simulink model "Innerloop_joystick_PIL_block"  (R2015a)
settings: Solver=ode45  StartTime=0.0  StopTime=100  FixedStep=0.01  RelTol=1e-3
undefined symbols (not defined in the file or in its folder): kdp, kdps, kdt, kdz, kpp, kpps, kpt, kpz
libraries: vrlib x1
settings Model: Creator=abdelrazzak.merheb  LastModifiedBy=flying
settings DataIOCC: SignalLoggingSaveFormat=ModelDataLogs
settings OptimizationCC: ExpressionDepthLimit=2147483647
settings DebuggingCC: UnderspecifiedInitializationDetection=Classic  MergeDetectMultiDrivingBlocksExec=none  SolverPrmCheckMsg=warning  FcnCallInpInsideContextMsg=UseLocalSettings  StateNameClashWarn=warning
settings GRTTargetCC: CombineOutputUpdateFcns=off  GRTInterface=on

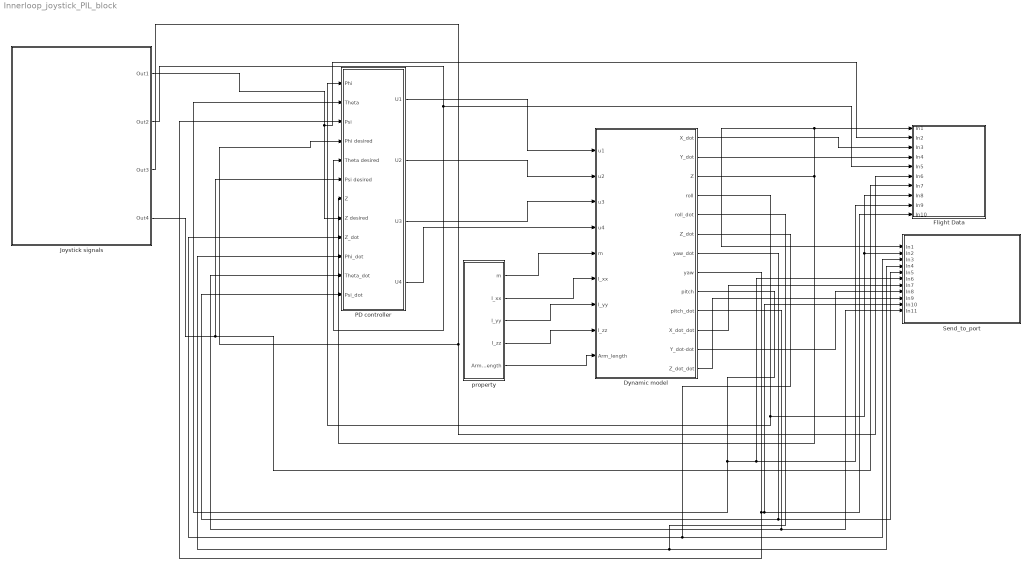
== system Innerloop_joystick_PIL_block ==
  Dynamic model : Subsystem
  Flight Data : Subsystem
  Joystick signals : Subsystem
  PD controller : Subsystem
  Send_to_port : Subsystem
  "property " : Subsystem
  wires:
  Dynamic model/9(pitch) -> PD controller/2(Theta), Flight Data/9(In9), Send_to_port/6(In6)
  Dynamic model/3(Z) -> PD controller/7(Z), Send_to_port/1(In1), Flight Data/1(In1)
  Dynamic model/4(roll) -> PD controller/1(Phi), Flight Data/8(In8), Send_to_port/2(In2)
  Dynamic model/6(Z_dot) -> Send_to_port/3(In3), PD controller/9(Z_dot)
  Dynamic model/5(roll_dot) -> Send_to_port/4(In4), PD controller/10(Phi_dot)
  Dynamic model/10(pitch_dot) -> PD controller/11(Theta_dot), Send_to_port/11(In11)
  Dynamic model/7(yaw_dot) -> PD controller/12("Psi_dot "), Send_to_port/5(In5)
  Dynamic model/8(yaw) -> PD controller/3(Psi), Flight Data/10(In10), Send_to_port/10(In10)
  Dynamic model/11(X_dot_dot) -> Send_to_port/7(In7)
  Dynamic model/12(Y_dot-dot) -> Send_to_port/8(In8)
  Dynamic model/13(Z_dot_dot) -> Send_to_port/9(In9)
  Joystick signals/4(Out4) -> Flight Data/7(In7), PD controller/6(Psi desired)
  Joystick signals/3(Out3) -> Flight Data/6(In6), PD controller/4(Phi desired)
  Joystick signals/2(Out2) -> PD controller/5(Theta desired), Flight Data/5(In5)
  Joystick signals/1(Out1) -> Flight Data/2(In2), PD controller/8(Z desired)
  Dynamic model/1("X_dot ") -> Flight Data/3(In3)
  Dynamic model/2(Y_dot) -> Flight Data/4(In4)
  "property "/5("Arm_length ") -> Dynamic model/9(Arm_length)
  "property "/4(I_zz) -> Dynamic model/8(I_zz)
  "property "/3(I_yy) -> Dynamic model/7(I_yy)
  "property "/2(I_xx) -> Dynamic model/6(I_xx)
  "property "/1(m) -> Dynamic model/5(m)
  PD controller/2(U2) -> Dynamic model/2(u2)
  PD controller/3(U3) -> Dynamic model/3(u3)
  PD controller/1(U1) -> Dynamic model/1(u1)
  PD controller/4(U4) -> Dynamic model/4(u4)

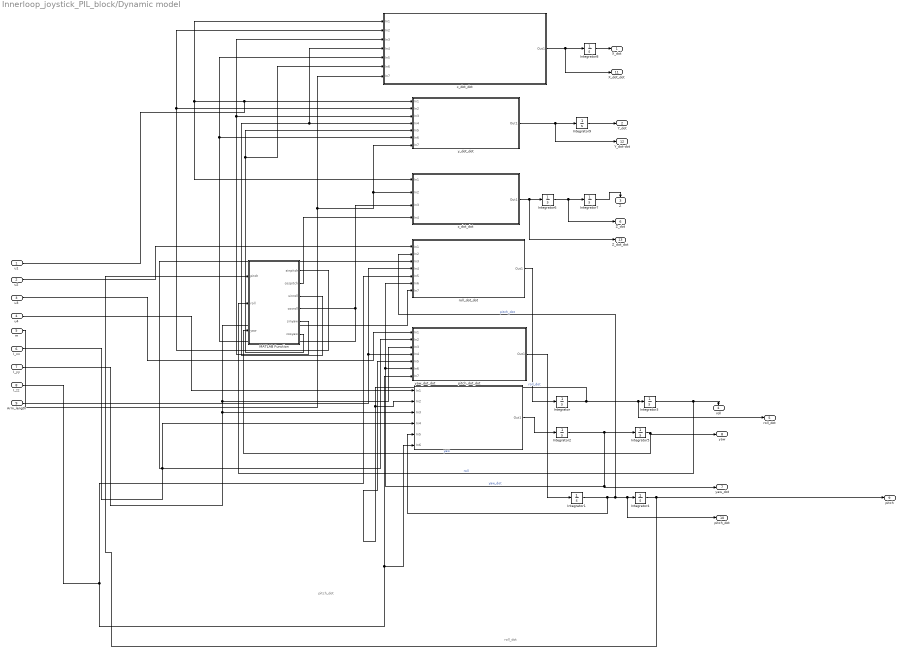
== system Innerloop_joystick_PIL_block/Dynamic model ==
  note: pitch_dot
  note: roll_dot
  u1 : Inport
  u2 : Inport  Port=2
  u3 : Inport  Port=3
  u4 : Inport  Port=4
  m : Inport  Port=5
  I_xx : Inport  Port=6
  I_yy : Inport  Port=7
  I_zz : Inport  Port=8
  Arm_length : Inport  Port=9
  Integrator{,1..9} (10 alike) : Integrator
  MATLAB Function : MATLAB Function  TreatAsAtomicUnit=on
  pitch_dot_dot : Subsystem
  roll_dot_dot : Subsystem
  x_dot_dot : Subsystem
  y_dot_dot : Subsystem
  yaw_dot_dot : Subsystem
  z_dot_dot : Subsystem
  "X_dot " : Outport
  Y_dot : Outport  Port=2
  Z : Outport  Port=3
  roll : Outport  Port=4
  roll_dot : Outport  Port=5
  Z_dot : Outport  Port=6
  yaw_dot : Outport  Port=7
  yaw : Outport  Port=8
  pitch : Outport  Port=9
  pitch_dot : Outport  Port=10
  X_dot_dot : Outport  Port=11
  Y_dot-dot : Outport  Port=12
  Z_dot_dot : Outport  Port=13
  wires:
  x_dot_dot/1(Out1) -> X_dot_dot/1, Integrator8/1
  Integrator6/1 -> Integrator7/1, Z_dot/1
  u4/1 -> yaw_dot_dot/1(In1)
  MATLAB Function/6(cosyaw) -> x_dot_dot/6(In6), y_dot_dot/5(In5)
  MATLAB Function/3(sinroll) -> x_dot_dot/4(In4), y_dot_dot/4(In4)
  MATLAB Function/4(cosroll) -> x_dot_dot/5(In5), y_dot_dot/6(In6), z_dot_dot/3(In3)
  MATLAB Function/1(sinpitch) -> x_dot_dot/2(In2), y_dot_dot/2(In2)
  m/1 -> x_dot_dot/7(In7), z_dot_dot/2(In2), y_dot_dot/7(In7)
  MATLAB Function/5(sinyaw) -> x_dot_dot/3(In3), y_dot_dot/3(In3)
  u1/1 -> y_dot_dot/1(In1), x_dot_dot/1(In1), z_dot_dot/1(In1)
  I_xx/1 -> yaw_dot_dot/4(In4), roll_dot_dot/3(In3), pitch_dot_dot/2(In2)
  I_yy/1 -> yaw_dot_dot/3(In3), roll_dot_dot/7(In7), pitch_dot_dot/3(In3)
  I_zz/1 -> roll_dot_dot/5(In5), yaw_dot_dot/6(In6), pitch_dot_dot/7(In7)
  Integrator3/1 -> roll/1, MATLAB Function/2(roll)  "roll"
  Integrator1/1 -> yaw_dot_dot/5(In5), roll_dot_dot/2(In2), pitch_dot/1, Integrator4/1  "pitch_dot"
  Integrator2/1 -> roll_dot_dot/6(In6), pitch_dot_dot/6(In6), yaw_dot/1, Integrator5/1  "yaw_dot"
  Integrator/1 -> pitch_dot_dot/5(In5), yaw_dot_dot/2(In2), roll_dot/1, Integrator3/1  "roll_dot"
  Integrator8/1 -> "X_dot "/1
  Integrator9/1 -> Y_dot/1
  Integrator5/1 -> MATLAB Function/3(yaw), yaw/1  "yaw"
  z_dot_dot/1(Out1) -> Z_dot_dot/1, Integrator6/1
  roll_dot_dot/1(Out1) -> Integrator/1
  pitch_dot_dot/1(Out1) -> Integrator1/1
  MATLAB Function/2(cospitch) -> z_dot_dot/4(In4)
  u2/1 -> roll_dot_dot/1(In1)
  Arm_length/1 -> roll_dot_dot/4(In4), pitch_dot_dot/4(In4)
  u3/1 -> pitch_dot_dot/1(In1)
  y_dot_dot/1(Out1) -> Y_dot-dot/1, Integrator9/1
  Integrator4/1 -> pitch/1, MATLAB Function/1(pitch)
  Integrator7/1 -> Z/1
  yaw_dot_dot/1(Out1) -> Integrator2/1

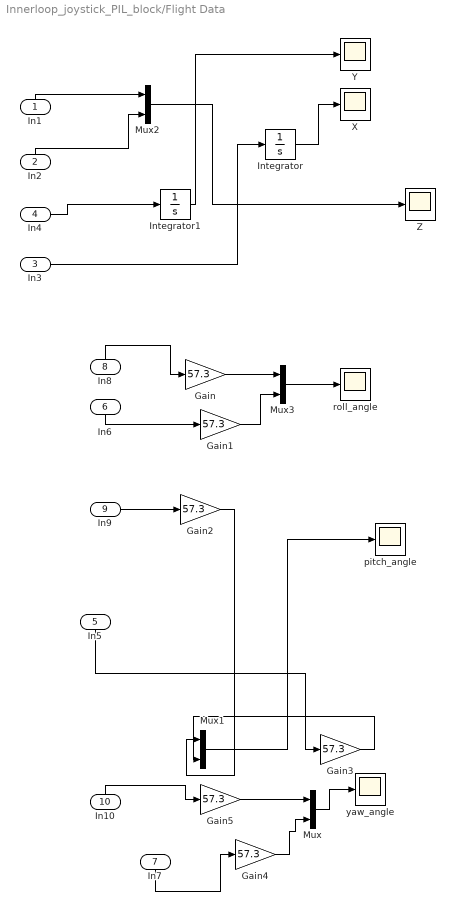
== system Innerloop_joystick_PIL_block/Flight Data ==
  In1 : Inport
  In2 : Inport  Port=2
  In3 : Inport  Port=3
  In4 : Inport  Port=4
  In5 : Inport  Port=5
  In6 : Inport  Port=6
  In7 : Inport  Port=7
  In8 : Inport  Port=8
  In9 : Inport  Port=9
  In10 : Inport  Port=10
  Gain{,1..5} (6 alike) : Gain  Gain=57.3
  Integrator : Integrator
  Integrator1 : Integrator
  Mux{,1..3} (4 alike) : Mux  Inputs=2
  X : Scope
      settings: YMin=-220  YMax=-160
  Y : Scope
      settings: YMin=-53000  YMax=-50750  SaveName=ScopeData2
  Z : Scope
      settings: YMin=95  YMax=105  SaveName=ScopeData3
  pitch_angle : Scope
  roll_angle : Scope
      settings: YMin=-7  YMax=12  SaveName=ScopeData4
  yaw_angle : Scope
      settings: YMin=2.5  YMax=8.5  SaveName=ScopeData5
  wires:
  In2/1 -> Mux2/2
  In1/1 -> Mux2/1
  In10/1 -> Gain5/1
  In9/1 -> Gain2/1
  In6/1 -> Gain1/1
  In7/1 -> Gain4/1
  In5/1 -> Gain3/1
  In8/1 -> Gain/1
  In4/1 -> Integrator1/1
  In3/1 -> Integrator/1
  Gain/1 -> Mux3/1
  Gain4/1 -> Mux/2
  Mux2/1 -> Z/1
  Gain5/1 -> Mux/1
  Mux1/1 -> pitch_angle/1
  Gain2/1 -> Mux1/1
  Gain3/1 -> Mux1/2
  Mux/1 -> yaw_angle/1
  Mux3/1 -> roll_angle/1
  Integrator1/1 -> Y/1
  Gain1/1 -> Mux3/2
  Integrator/1 -> X/1

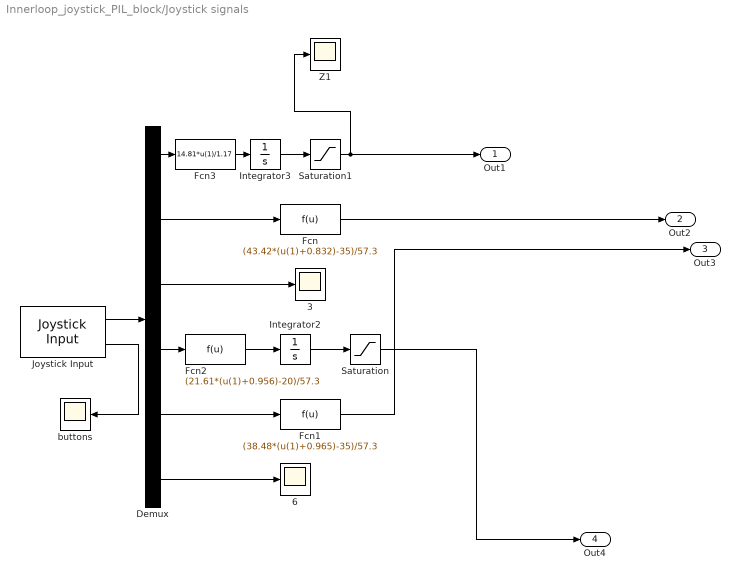
== system Innerloop_joystick_PIL_block/Joystick signals ==
  3 : Scope
      settings: SaveName=ScopeData9
  6 : Scope
      settings: SaveName=ScopeData10
  Demux : Demux  Outputs=6
  Fcn : Fcn  Expr=(43.42*(u(1)+0.832)-35)/57.3
  Fcn1 : Fcn  Expr=(38.48*(u(1)+0.965)-35)/57.3
  Fcn2 : Fcn  Expr=(21.61*(u(1)+0.956)-20)/57.3
  Fcn3 : Fcn  Expr=14.81*u(1)/1.17
  Integrator2 : Integrator
  Integrator3 : Integrator
  Joystick Input : vrlib/Joystick Input  joyid=1  adjustports=on  forcefeed=off
  Saturation : Saturate  UpperLimit=pi  LowerLimit=-pi
  Saturation1 : Saturate  UpperLimit=100  LowerLimit=0
  Z1 : Scope
      settings: YMin=-0.774  YMax=-0.765  SaveName=ScopeData7
  buttons : Scope
      settings: SaveName=ScopeData12
  Out1 : Outport
  Out2 : Outport  Port=2
  Out3 : Outport  Port=3
  Out4 : Outport  Port=4
  wires:
  Integrator2/1 -> Saturation/1
  Joystick Input/1 -> Demux/1
  Demux/1 -> Fcn3/1
  Demux/3 -> 3/1
  Demux/5 -> Fcn1/1
  Demux/2 -> Fcn/1
  Demux/6 -> 6/1
  Joystick Input/2 -> buttons/1
  Demux/4 -> Fcn2/1
  Fcn3/1 -> Integrator3/1
  Integrator3/1 -> Saturation1/1
  Fcn/1 -> Out2/1
  Fcn1/1 -> Out3/1
  Saturation/1 -> Out4/1
  Saturation1/1 -> Out1/1, Z1/1
  Fcn2/1 -> Integrator2/1

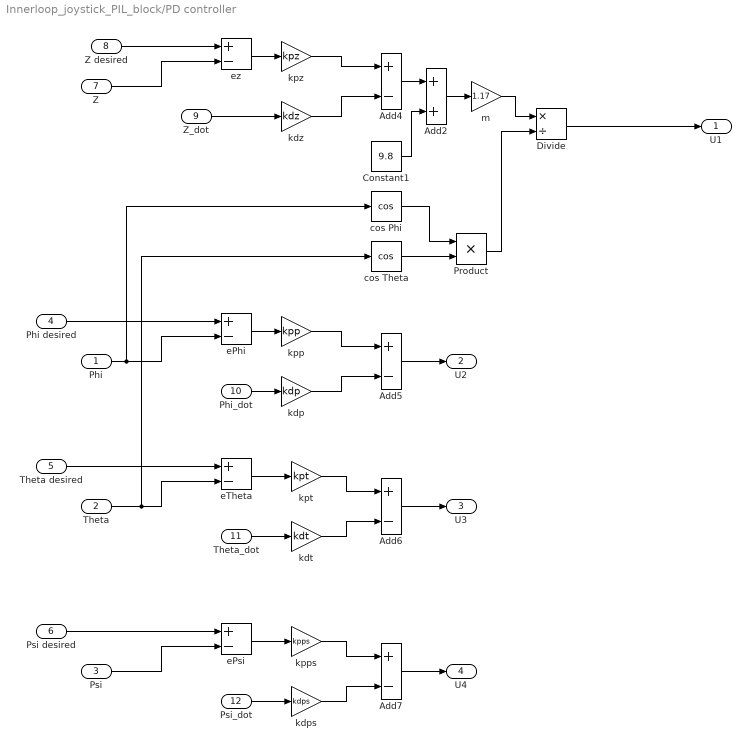
== system Innerloop_joystick_PIL_block/PD controller ==
  Phi : Inport
  Theta : Inport  Port=2
  Psi : Inport  Port=3
  Phi desired : Inport  Port=4
  Theta desired : Inport  Port=5
  Psi desired : Inport  Port=6
  Z : Inport  Port=7
  Z desired : Inport  Port=8
  Z_dot : Inport  Port=9
  Phi_dot : Inport  Port=10
  Theta_dot : Inport  Port=11
  "Psi_dot " : Inport  Port=12
  Add2 : Sum
  Add{4..7} (4 alike) : Sum  Inputs=+-
  Constant1 : Constant  Value=9.8
  Divide : Product  Inputs=*/
  Product : Product  RndMeth=Zero
  cos Phi : Trigonometry  Operator=cos
  cos Theta : Trigonometry  Operator=cos
  ePhi : Sum  Inputs=+-
  ePsi : Sum  Inputs=+-
  eTheta : Sum  Inputs=+-
  ez : Sum  Inputs=+-
  kdp : Gain  Gain=kdp
  kdps : Gain  Gain=kdps
  kdt : Gain  Gain=kdt
  kdz : Gain  Gain=kdz
  kpp : Gain  Gain=kpp
  kpps : Gain  Gain=kpps
  kpt : Gain  Gain=kpt
  kpz : Gain  Gain=kpz
  m : Gain  Gain=1.17
  U1 : Outport
  U2 : Outport  Port=2
  U3 : Outport  Port=3
  U4 : Outport  Port=4
  wires:
  Phi/1 -> ePhi/2, cos Phi/1
  Theta/1 -> eTheta/2, cos Theta/1
  Psi/1 -> ePsi/2
  Phi desired/1 -> ePhi/1
  Theta desired/1 -> eTheta/1
  Psi desired/1 -> ePsi/1
  ePhi/1 -> kpp/1
  Phi_dot/1 -> kdp/1
  eTheta/1 -> kpt/1
  Theta_dot/1 -> kdt/1
  ePsi/1 -> kpps/1
  "Psi_dot "/1 -> kdps/1
  Z desired/1 -> ez/1
  ez/1 -> kpz/1
  Z_dot/1 -> kdz/1
  kpz/1 -> Add4/1
  kdz/1 -> Add4/2
  kpp/1 -> Add5/1
  kdp/1 -> Add5/2
  Add5/1 -> U2/1
  kpt/1 -> Add6/1
  kdt/1 -> Add6/2
  Add6/1 -> U3/1
  kpps/1 -> Add7/1
  kdps/1 -> Add7/2
  Add7/1 -> U4/1
  cos Phi/1 -> Product/1
  cos Theta/1 -> Product/2
  m/1 -> Divide/1
  Product/1 -> Divide/2
  Divide/1 -> U1/1
  Add4/1 -> Add2/1
  Add2/1 -> m/1
  Constant1/1 -> Add2/2
  Z/1 -> ez/2

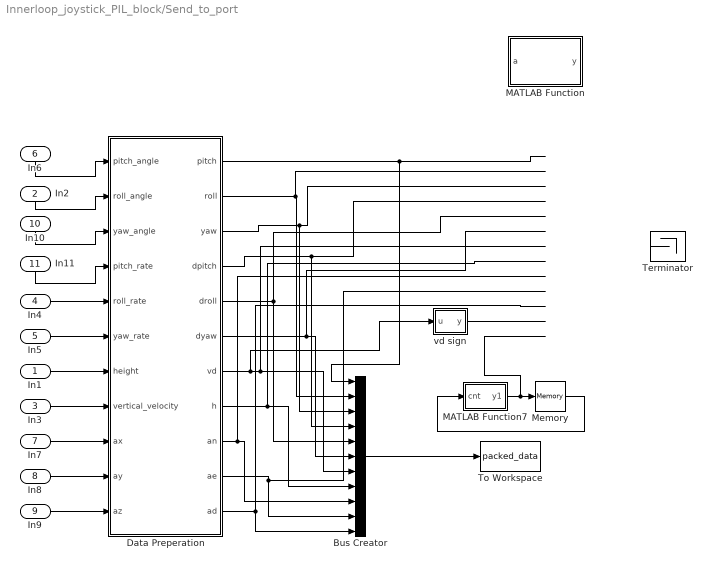
== system Innerloop_joystick_PIL_block/Send_to_port ==
  In1 : Inport
  In2 : Inport  Port=2
  In3 : Inport  Port=3
  In4 : Inport  Port=4
  In5 : Inport  Port=5
  In6 : Inport  Port=6
  In7 : Inport  Port=7
  In8 : Inport  Port=8
  In9 : Inport  Port=9
  In10 : Inport  Port=10
  In11 : Inport  Port=11
  Bus Creator : BusCreator  Inputs=11
  Data Preperation : MATLAB Function  TreatAsAtomicUnit=on
  MATLAB Function : MATLAB Function  TreatAsAtomicUnit=on
  MATLAB Function7 : MATLAB Function  TreatAsAtomicUnit=on
  Memory : Memory
  Terminator : Terminator
  To Workspace : ToWorkspace  VariableName=packed_data  SampleTime=-1
      settings: Save2DSignal=2-D array (concatenate along first dimension)
  vd sign : MATLAB Function  TreatAsAtomicUnit=on
  wires:
  Data Preperation/5(droll) -> Bus Creator/5
  Data Preperation/10(ae) -> Bus Creator/10
  In7/1 -> Data Preperation/9(ax)
  Data Preperation/6(dyaw) -> Bus Creator/6
  Data Preperation/7(vd) -> vd sign/1(u), Bus Creator/7
  Data Preperation/8(h) -> Bus Creator/8
  Bus Creator/1 -> To Workspace/1
  Data Preperation/3(yaw) -> Bus Creator/3
  Data Preperation/9(an) -> Bus Creator/9
  Data Preperation/4(dpitch) -> Bus Creator/4
  vd sign/1(y) -> ?
  MATLAB Function7/1(y1) -> Memory/1
  Data Preperation/2(roll) -> Bus Creator/2
  ? -> Terminator/1
  In8/1 -> Data Preperation/10(ay)
  Data Preperation/11(ad) -> Bus Creator/11
  Data Preperation/1(pitch) -> Bus Creator/1
  In9/1 -> Data Preperation/11(az)
  Memory/1 -> MATLAB Function7/1(cnt)
  In5/1 -> Data Preperation/6(yaw_rate)
  In1/1 -> Data Preperation/7(height)
  In10/1 -> Data Preperation/3(yaw_angle)
  In6/1 -> Data Preperation/1(pitch_angle)
  In4/1 -> Data Preperation/5(roll_rate)
  In11/1 -> Data Preperation/4(pitch_rate)
  In3/1 -> Data Preperation/8(vertical_velocity)
  In2/1 -> Data Preperation/2(roll_angle)

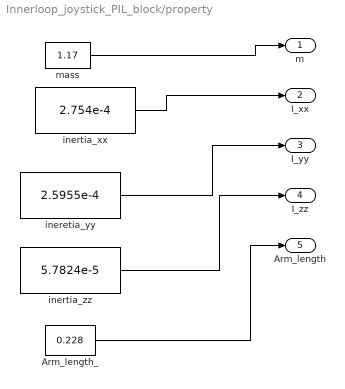
== system Innerloop_joystick_PIL_block/property  ==
  Arm_length_ : Constant  Value=0.228
  ineretia_yy : Constant  Value=2.5955e-4
  inertia_xx : Constant  Value=2.754e-4
  inertia_zz : Constant  Value=5.7824e-5
  mass : Constant  Value=1.17
  m : Outport
  I_xx : Outport  Port=2
  I_yy : Outport  Port=3
  I_zz : Outport  Port=4
  "Arm_length " : Outport  Port=5
  wires:
  inertia_zz/1 -> I_zz/1
  Arm_length_/1 -> "Arm_length "/1
  ineretia_yy/1 -> I_yy/1
  mass/1 -> m/1
  inertia_xx/1 -> I_xx/1

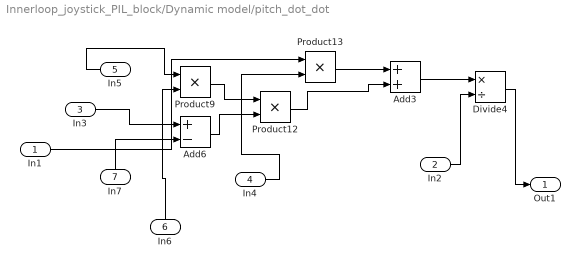
== system Innerloop_joystick_PIL_block/Dynamic model/pitch_dot_dot ==
  In1 : Inport
  In2 : Inport  Port=2
  In3 : Inport  Port=3
  In4 : Inport  Port=4
  In5 : Inport  Port=5
  In6 : Inport  Port=6
  In7 : Inport  Port=7
  Add3 : Sum
  Add6 : Sum  Inputs=+-
  Divide4 : Product  Inputs=*/
  Product12 : Product
  Product13 : Product
  Product9 : Product
  Out1 : Outport
  wires:
  Product12/1 -> Add3/2
  Product13/1 -> Add3/1
  In1/1 -> Product13/1
  Add6/1 -> Product12/2
  Add3/1 -> Divide4/1
  Product9/1 -> Product12/1
  In4/1 -> Product13/2
  In6/1 -> Product9/2
  In7/1 -> Add6/2
  In3/1 -> Add6/1
  In2/1 -> Divide4/2
  In5/1 -> Product9/1
  Divide4/1 -> Out1/1

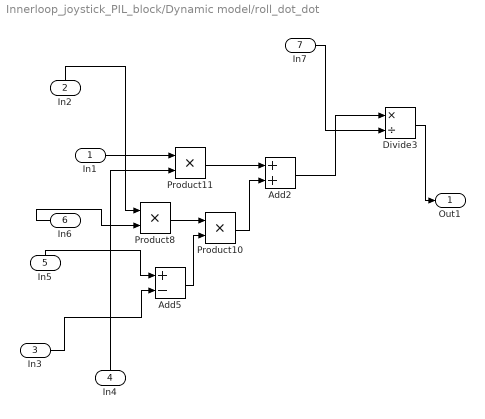
== system Innerloop_joystick_PIL_block/Dynamic model/roll_dot_dot ==
  In1 : Inport
  In2 : Inport  Port=2
  In3 : Inport  Port=3
  In4 : Inport  Port=4
  In5 : Inport  Port=5
  In6 : Inport  Port=6
  In7 : Inport  Port=7
  Add2 : Sum
  Add5 : Sum  Inputs=+-
  Divide3 : Product  Inputs=*/
  Product10 : Product
  Product11 : Product
  Product8 : Product
  Out1 : Outport
  wires:
  Product11/1 -> Add2/1
  Add5/1 -> Product10/2
  In1/1 -> Product11/1
  Add2/1 -> Divide3/1
  Product8/1 -> Product10/1
  Product10/1 -> Add2/2
  Divide3/1 -> Out1/1
  In5/1 -> Add5/1
  In3/1 -> Add5/2
  In2/1 -> Product8/1
  In7/1 -> Divide3/2
  In4/1 -> Product11/2
  In6/1 -> Product8/2

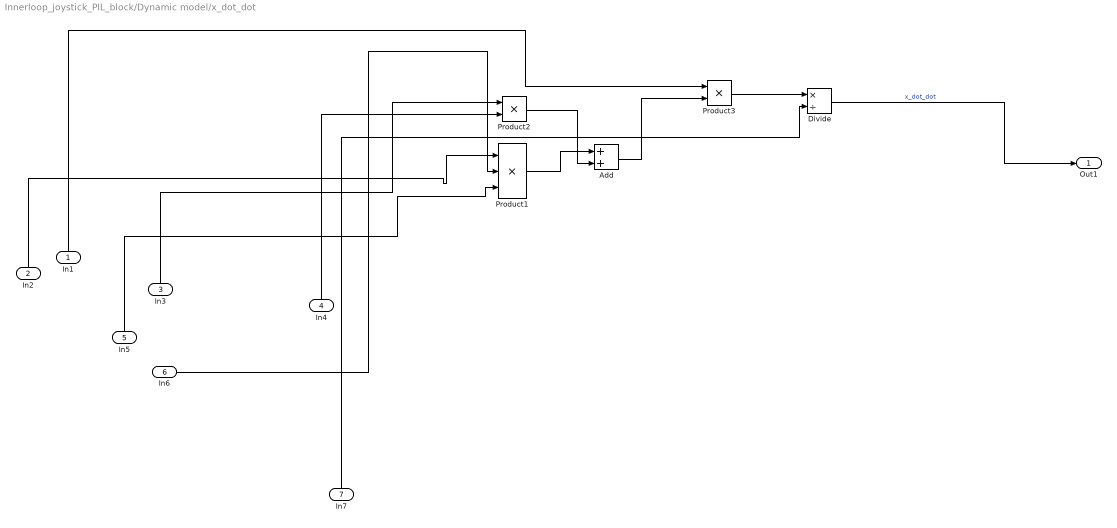
== system Innerloop_joystick_PIL_block/Dynamic model/x_dot_dot ==
  In1 : Inport
  In2 : Inport  Port=2
  In3 : Inport  Port=3
  In4 : Inport  Port=4
  In5 : Inport  Port=5
  In6 : Inport  Port=6
  In7 : Inport  Port=7
  Add : Sum
  Divide : Product  Inputs=*/
  Product1 : Product  Inputs=3
  Product2 : Product
  Product3 : Product
  Out1 : Outport
  wires:
  In1/1 -> Product3/1
  In6/1 -> Product1/2
  In7/1 -> Divide/2
  In4/1 -> Product2/2
  In3/1 -> Product2/1
  In5/1 -> Product1/3
  In2/1 -> Product1/1
  Divide/1 -> Out1/1  "x_dot_dot"
  Product2/1 -> Add/2
  Product1/1 -> Add/1
  Product3/1 -> Divide/1
  Add/1 -> Product3/2

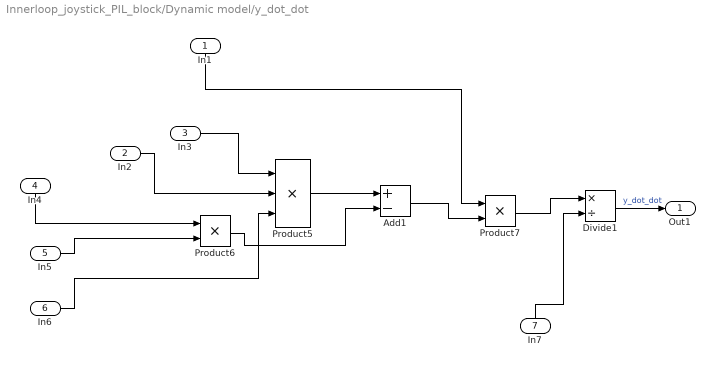
== system Innerloop_joystick_PIL_block/Dynamic model/y_dot_dot ==
  In1 : Inport
  In2 : Inport  Port=2
  In3 : Inport  Port=3
  In4 : Inport  Port=4
  In5 : Inport  Port=5
  In6 : Inport  Port=6
  In7 : Inport  Port=7
  Add1 : Sum  Inputs=+-
  Divide1 : Product  Inputs=*/
  Product5 : Product  Inputs=3
  Product6 : Product
  Product7 : Product
  Out1 : Outport
  wires:
  In1/1 -> Product7/1
  In2/1 -> Product5/2
  In5/1 -> Product6/2
  In7/1 -> Divide1/2
  In6/1 -> Product5/3
  In3/1 -> Product5/1
  In4/1 -> Product6/1
  Product5/1 -> Add1/1
  Add1/1 -> Product7/2
  Product6/1 -> Add1/2
  Divide1/1 -> Out1/1  "y_dot_dot"
  Product7/1 -> Divide1/1

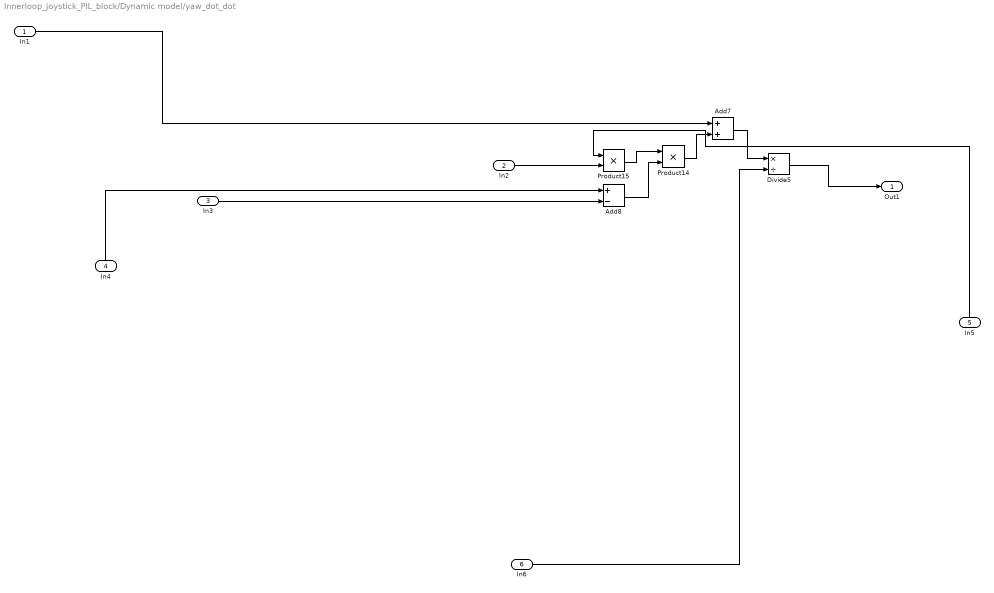
== system Innerloop_joystick_PIL_block/Dynamic model/yaw_dot_dot ==
  In1 : Inport
  In2 : Inport  Port=2
  In3 : Inport  Port=3
  In4 : Inport  Port=4
  In5 : Inport  Port=5
  In6 : Inport  Port=6
  Add7 : Sum
  Add8 : Sum  Inputs=+-
  Divide5 : Product  Inputs=*/
  Product14 : Product
  Product15 : Product
  Out1 : Outport
  wires:
  In4/1 -> Add8/1
  In6/1 -> Divide5/2
  In2/1 -> Product15/2
  In3/1 -> Add8/2
  In5/1 -> Product15/1
  Product14/1 -> Add7/2
  Add8/1 -> Product14/2
  Product15/1 -> Product14/1
  In1/1 -> Add7/1
  Add7/1 -> Divide5/1
  Divide5/1 -> Out1/1

== system Innerloop_joystick_PIL_block/Dynamic model/z_dot_dot ==
  In1 : Inport
  In2 : Inport  Port=2
  In3 : Inport  Port=3
  In4 : Inport  Port=4
  Add4 : Sum  Inputs=-+
  Divide2 : Product  Inputs=*/
  Product : Product
  Product4 : Product
  u5 : Constant  Value=9.8
  Out1 : Outport
  wires:
  In3/1 -> Product4/2
  In2/1 -> Divide2/2
  In1/1 -> Product/2
  Divide2/1 -> Add4/2
  Product4/1 -> Product/1
  In4/1 -> Product4/1
  u5/1 -> Add4/1
  Product/1 -> Divide2/1
  Add4/1 -> Out1/1  "z_dot_dot"

== matlab function Innerloop_joystick_PIL_block/Send_to_port/vd sign ==
  data: u input; y output
function y = fcn(u)
if u>0;
y=bin2dec('00000000');
elseif u==0
y=bin2dec('00000000');
else u<0;
y=bin2dec('00000100');
end

== matlab function Innerloop_joystick_PIL_block/Send_to_port/Data Preperation ==
  data: pitch output; roll output; yaw output; pitch_angle input; roll_angle input; yaw_angle input; pitch_rate input; roll_rate input; yaw_rate input; dpitch output; droll output; dyaw output; vd output; h output; height input; an output; ae output; ad output; vertical_velocity input; ax input; ay input; az input
function [pitch,roll,yaw,dpitch,droll,dyaw,vd,h,an,ae,ad] = fcn(pitch_angle,roll_angle,yaw_angle,pitch_rate,roll_rate,yaw_rate,height,vertical_velocity,ax,ay,az)

pitch=round(pitch_angle*573);
roll=round(roll_angle*573);
yaw=round(yaw_angle*573);


dpitch=round(pitch_rate*573);
droll=round(roll_rate*573);
dyaw=round(yaw_rate*573);


h=round(height*1000);
vd=round(vertical_velocity*100);


Rotation_metrix=[
                  cos(pitch_angle)*cos(yaw_angle)-cos(roll_angle)*sin(pitch_angle)*sin(yaw_angle),-cos(roll_angle)*cos(yaw_angle)*sin(pitch_angle)-cos(pitch_angle)*sin(yaw_angle),sin(pitch_angle)*sin(roll_angle);
                  cos(yaw_angle)*sin(pitch_angle)+cos(pitch_angle)*cos(roll_angle)*sin(yaw_angle),cos(pitch_angle)*cos(roll_angle)-sin(pitch_angle)*sin(yaw_angle),-cos(pitch_angle)*sin(roll_angle);
                  sin(roll_angle)*sin(yaw_angle),cos(yaw_angle)*sin(roll_angle),cos(roll_angle)
];

B=[ax,ay,az]';
A=Rotation_metrix*B;
an=A(1,1);
ae=A(2,1);
ad=A(3,1);

an=round(an*100);
ae=round(ae*100);
ad=round(ad*100);

== matlab function Innerloop_joystick_PIL_block/Send_to_port/MATLAB Function ==
  data: y output; a input
function y = fcn(a)

a=a*2;
IMU_data_pack=zeros(1,41);

IMU_data_pack(1,1)=165;%帧头
IMU_data_pack(1,2)=90;%帧头
IMU_data_pack(1,3)=83;%帧长度
IMU_data_pack(1,4)=0;%保留
IMU_data_pack(1,5)=97;%帧标志
%数据段
IMU_data_pack(1,6)=127;%Flag0
IMU_data_pack(1,7)=11;%Flag1
IMU_data_pack(1,8)=128;%NavStatus
IMU_data_1_8=[IMU_data_pack(1,1),IMU_data_pack(1,2),IMU_data_pack(1,3),IMU_data_pack(1,4),IMU_data_pack(1,5),IMU_data_pack(1,6),    IMU_data_pack(1,7),IMU_data_pack(1,8)];

% Pitch,Roll,Yaw
IMU_data_pack(1,9)=-1;%block.InputPort(1).Data; %0,1
IMU_data_pack(1,10)=-1;%block.InputPort(2).Data;%2,3
IMU_data_pack(1,11)=-1;%block.InputPort(3).Data;%4,5
IMU_data_9_10_11=[IMU_data_pack(1,9),IMU_data_pack(1,10),IMU_data_pack(1,11)];
%q0,q1,q2,q3
IMU_data_pack(1,12)=-1;%6,7,8,9
IMU_data_pack(1,13)=-1;%10,11,12,13
IMU_data_pack(1,14)=-1;%14,15,16,17
IMU_data_pack(1,15)=-1;%18,19,20,21
IMU_data_12_13_14_15=[IMU_data_pack(1,12),IMU_data_pack(1,13),IMU_data_pack(1,14),IMU_data_pack(1,15)];
%dpitch,droll,dyaw 22~27
IMU_data_pack(1,16)= -1;%block.InputPort(4).Data;
IMU_data_pack(1,17)= -1;%block.InputPort(5).Data;
IMU_data_pack(1,18)=-1;% block.InputPort(6).Data;
IMU_data_9_10_11=[IMU_data_pack(1,16),IMU_data_pack(1,17),IMU_data_pack(1,18)];
%AngRateN,AngRateE,AngRateD 28~33
IMU_data_pack(1,19)=257;
IMU_data_pack(1,20)=257;
IMU_data_pack(1,21)=257;
IMU_data_19_20_21=[IMU_data_pack(1,19),IMU_data_pack(1,20),IMU_data_pack(1,21)];
%AngRateX,AngRateY,AngRateZ 34~39
IMU_data_pack(1,22)=258;
IMU_data_pack(1,23)=258;
IMU_data_pack(1,24)=258;
IMU_data_22_23_24=[IMU_data_pack(1,22),IMU_data_pack(1,23),IMU_data_pack(1,24)];
%Position 40~51
IMU_data_pack(1,25)=-1;
IMU_data_pack(1,26)=-1;
IMU_data_pack(1,27)=-1;%block.InputPort(8).Data;
IMU_data_25_26_27=[IMU_data_pack(1,25),IMU_data_pack(1,26),IMU_data_pack(1,27)];
%Velocity NED
IMU_data_pack(1,28)=1;%block.InputPort(12).Data; 52
%53~58
IMU_data_pack(1,29)=259;
IMU_data_pack(1,30)=259;
IMU_data_pack(1,31)=259;%block.InputPort(7).Data;
IMU_data_29_30_31=[IMU_data_pack(1,29),IMU_data_pack(1,30),IMU_data_pack(1,31)];
%Acceleration NED 59~64
IMU_data_pack(1,32)=-1;%block.InputPort(9).Data;
IMU_data_pack(1,33)=-1;%block.InputPort(10).Data;
IMU_data_pack(1,34)=-1;%block.InputPort(11).Data;
IMU_data_32_33_34=[IMU_data_pack(1,32),IMU_data_pack(1,33),IMU_data_pack(1,34)];
%Acceleration XYZ 65~70
IMU_data_pack(1,35)=257;
IMU_data_pack(1,36)=257;
IMU_data_pack(1,37)=258;
IMU_data_35_36_37=[IMU_data_pack(1,35),IMU_data_pack(1,36),IMU_data_pack(1,37)];
%AirHeight 71~74
IMU_data_pack(1,38)=-1;%block.InputPort(8).Data;
%cnt
cnt=1;%block.InputPort(13).Data;
IMU_data_pack(1,39)=cnt;%block.InputPort(13).Data;

%%%%%%%%%%%%%Split Data for CRC 1~84
IMU_split_crc=zeros(1,86);
%1~8
j=1;
for i=1:1:8
IMU_split_crc(1,i)=IMU_data_pack(1,i);
j=j+1;
end
%9~14 pitch,roll,yaw
for i=9:1:11
    a=dec_to_bia(IMU_data_pack(1,i),16);    
   IMU_split_crc(1,j)=bin2dec(a(9:16));
   j=j+1;
   IMU_split_crc(1,j)=bin2dec(a(1:8));
   j=j+1;
end
%15~30 q0,q1,q2,q3
for i=12:1:15
    a=dec_to_bia(IMU_data_pack(1,i),32);
    IMU_split_crc(1,j)=bin2dec(a(25:32));
    j=j+1;
    IMU_split_crc(1,j)=bin2dec(a(17:24));
    j=j+1;
    IMU_split_crc(1,j)=bin2dec(a(9:16));
    j=j+1;
    IMU_split_crc(1,j)=bin2dec(a(1:8));
    j=j+1;
end
%31~36 dpitch,droll,dyaw
for i=16:1:18
a=dec_to_bia(IMU_data_pack(1,i),16);
IMU_split_crc(1,j)=bin2dec(a(9:16));
j=j+1;
IMU_split_crc(1,j)=bin2dec(a(1:8));
j=j+1;
end
%37~42 AngRateN,AngRateE,AngRateD
for i=19:1:21
a=dec_to_bia(IMU_data_pack(1,i),16);
IMU_split_crc(1,j)=bin2dec(a(9:16));
j=j+1;
IMU_split_crc(1,j)=bin2dec(a(1:8));
j=j+1;
end
%43~48 AngRateX,AngRateY,AngRateZ
for i=22:1:24
a=dec_to_bia(IMU_data_pack(1,i),16);
IMU_split_crc(1,j)=bin2dec(a(9:16));
j=j+1;
IMU_split_crc(1,j)=bin2dec(a(1:8));
j=j+1;
end
%49~60 X,Y,Z
for i=25:1:27
a=dec_to_bia(IMU_data_pack(1,i),32);
IMU_split_crc(1,j)=bin2dec(a(25:32));
j=j+1;
IMU_split_crc(1,j)=bin2dec(a(17:24));
j=j+1;
IMU_split_crc(1,j)=bin2dec(a(9:16));
j=j+1;
IMU_split_crc(1,j)=bin2dec(a(1:8));
j=j+1;
end
%61 sign
i=28;
a=dec_to_bia(IMU_data_pack(1,i),8);
IMU_split_crc(1,j)=bin2dec(a(1:8));
j=j+1;
%62~67 VN,VE,VD 
for i=29:1:31
a=dec_to_bia(IMU_data_pack(1,i),16);  
IMU_split_crc(1,j)=bin2dec(a(9:16));
j=j+1;
IMU_split_crc(1,j)=bin2dec(a(1:8));
j=j+1;
end
%68~73 an,ae,ad
for i=32:1:34
a=dec_to_bia(IMU_data_pack(1,i),16);  
IMU_split_crc(1,j)=bin2dec(a(9:16));
j=j+1;
IMU_split_crc(1,j)=bin2dec(a(1:8));
j=j+1;
end
%74~79 ax,ay,az
for i=35:1:37
a=dec_to_bia(IMU_data_pack(1,i),16);  
IMU_split_crc(1,j)=bin2dec(a(9:16));
j=j+1;
IMU_split_crc(1,j)=bin2dec(a(1:8));
j=j+1;
end
%80~83 height
i=38;
a=dec_to_bia(IMU_data_pack(1,i),32);
IMU_split_crc(1,j)=bin2dec(a(25:32));
j=j+1;
IMU_split_crc(1,j)=bin2dec(a(17:24));
j=j+1;
IMU_split_crc(1,j)=bin2dec(a(9:16));
j=j+1;
IMU_split_crc(1,j)=bin2dec(a(1:8));
j=j+1;
%84 cnt
i=39;
a=dec_to_bia(IMU_data_pack(1,i),8);
IMU_split_crc(1,j)=bin2dec(a(1:8));
%%%%%%%%%%%%%%%%%%%%%
%fwrite(s,IMU_split_crc(1,1:84),'uchar');
%CRC
crc_gen=uint16(40961);
crc=uint16(65535);
buf_len=84;
 if (buf_len~=0)
    for i=1:1:buf_len
        crc=uint16(bitxor(crc,uint16(IMU_split_crc(1,i))));
        for j=1:1:8;           
        if (bitand(crc,1)==1)
           crc=uint16(bitshift(crc,-1));
           crc=uint16(bitxor(crc,crc_gen));
       else
           crc=uint16(bitshift(crc,-1));
       end
        end
    end
 end
IMU_data_pack(1,40)=crc;

a=dec_to_bia(IMU_data_pack(1,40),16);
IMU_split_crc(1,85)=bin2dec(a(9:16));
IMU_split_crc(1,86)=bin2dec(a(1:8));


%checksum
checksum=0;
for j=1:1:86;    
    checksum_data=IMU_split_crc(1,j);     
    checksum=checksum_data+checksum;  
end


y =IMU_split_crc;

== matlab function Innerloop_joystick_PIL_block/Dynamic model/MATLAB Function ==
  data: pitch input; sinpitch output; roll input; yaw input; cospitch output; sinroll output; cosroll output; sinyaw output; cosyaw output
function [sinpitch,cospitch,sinroll,cosroll,sinyaw,cosyaw]= fcn(pitch,roll,yaw)
sinpitch=sin(pitch);
cospitch=cos(pitch);
sinroll=sin(roll);
cosroll=cos(roll);
sinyaw=sin(yaw);
cosyaw=cos(yaw);

== matlab function Innerloop_joystick_PIL_block/Send_to_port/MATLAB Function7 ==
  data: y1 output; cnt input
function y1= fcn(cnt)



y1=cnt+1;
if y1>255
y1=1;
end
